simulink model "SA_asservissement_seul"  (R2016a)
settings: Solver=VariableStepAuto  StartTime=0.0  StopTime=5  RelTol=1e-3
values from neighbouring files (symbols this model uses):
  den_a_Z = [1 -p]    [SA_9.m]    (also in SA_global.m)
  den_AvPh = [1 -p]    [SA_global.m]
  den_PI = [1 -p]    [SA_global.m]
  den_r_Z = [1 -p_re]    [SA_9.m]    (also in SA_global.m)
  Ka_SA8 = abs((polyval(den_phi,pdes)*polyval(den_AvPh_SA8,pdes)*polyval(den_PI_SA8,pdes))/(polyval(num_AvPh_SA8,pdes)*polyval(num_phi,pdes)*polyval(num_PI_SA8,pdes)))    [SA_8.m]    (also in SA_global.m = abs((polyval(den_phi,pdes)*polyval(den_AvPh,pdes)*polyval(de)
  Kp_XX = -z*Kv_XX    [SA_10.m]    (also in SA_10x.m; SA_10y.m; SA_global.m)
  Kp_YY = -z*Kv_YY    [SA_10y.m]    (also in SA_global.m)
  Kv_XX = 1/abs(polyval(conv(num_a_XX,num_Sx(1,:)),p_des)/polyval(conv(den_a_XX,den_Sx),p_des))    [SA_10.m]    (also in SA_10x.m; SA_10y.m; SA_global.m)
  Kv_YY = 1/abs(polyval(conv(num_a_YY,num_Sy(1,:)),p_des)/polyval(conv(den_a_YY,den_Sy),p_des))    [SA_10y.m]    (also in SA_global.m)
  num_a_Z = Ka_Z*[1 -z]    [SA_9.m]    (also in SA_global.m)
  num_AvPh = [1 -z]    [SA_global.m]
  num_PI = [1 -z]    [SA_global.m]
  num_r_Z = [1 -z_re]    [SA_9.m]    (also in SA_global.m)
undefined symbols (not defined in the file or in its folder): A_theta, A_z, B_theta, B_z, C_theta, C_z, D_theta_1sortie, D_z_1sortie
settings Model: Creator=genp2203  LastModifiedBy=genp2203

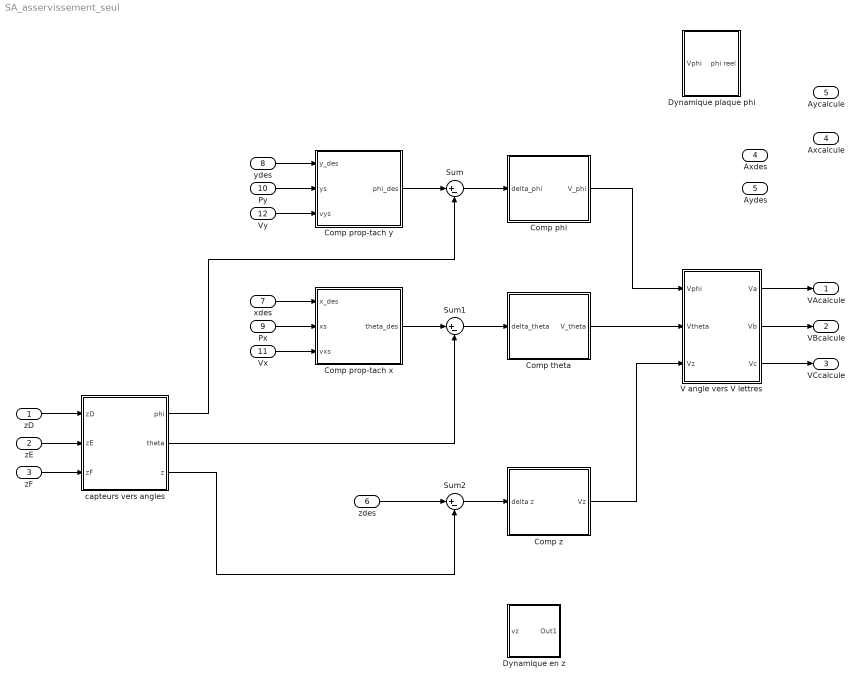
== system SA_asservissement_seul ==
  zD : Inport
  zE : Inport  Port=2
  zF : Inport  Port=3
  Axdes : Inport  Port=4
  Aydes : Inport  Port=5
  zdes : Inport  Port=6
  xdes : Inport  Port=7
  ydes : Inport  Port=8
  Px : Inport  Port=9
  Py : Inport  Port=10
  Vx : Inport  Port=11
  Vy : Inport  Port=12
  Comp phi : Subsystem
  Comp prop-tach x : Subsystem
  Comp prop-tach y : Subsystem
  Comp theta : Subsystem
  Comp z : Subsystem
  Dynamique en z : Subsystem
  Dynamique plaque phi : Subsystem
  Sum : Sum  Inputs=|+-
  Sum1 : Sum  Inputs=|+-
  Sum2 : Sum  Inputs=|+-
  V angle vers V lettres : Subsystem
  capteurs vers angles : Subsystem
  VAcalcule : Outport
  VBcalcule : Outport  Port=2
  VCcalcule : Outport  Port=3
  Axcalcule : Outport  Port=4
  Aycalcule : Outport  Port=5
  wires:
  Sum/1 -> Comp phi/1(delta_phi)
  ydes/1 -> Comp prop-tach y/1(y_des)
  xdes/1 -> Comp prop-tach x/1(x_des)
  Vx/1 -> Comp prop-tach x/3(vxs)
  Px/1 -> Comp prop-tach x/2(xs)
  Py/1 -> Comp prop-tach y/2(ys)
  Vy/1 -> Comp prop-tach y/3(vys)
  Comp prop-tach y/1(phi_des) -> Sum/1
  zD/1 -> capteurs vers angles/1(zD)
  zE/1 -> capteurs vers angles/2(zE)
  zF/1 -> capteurs vers angles/3(zF)
  capteurs vers angles/1(phi) -> Sum/2
  V angle vers V lettres/3(Vc) -> VCcalcule/1
  V angle vers V lettres/2(Vb) -> VBcalcule/1
  V angle vers V lettres/1(Va) -> VAcalcule/1
  Comp phi/1(V_phi) -> V angle vers V lettres/1(Vphi)
  Comp theta/1(V_theta) -> V angle vers V lettres/2(Vtheta)
  Comp prop-tach x/1(theta_des) -> Sum1/1
  Sum1/1 -> Comp theta/1(delta_theta)
  capteurs vers angles/2(theta) -> Sum1/2
  capteurs vers angles/3(z) -> Sum2/2
  zdes/1 -> Sum2/1
  Sum2/1 -> Comp z/1(delta z)
  Comp z/1(Vz) -> V angle vers V lettres/3(Vz)

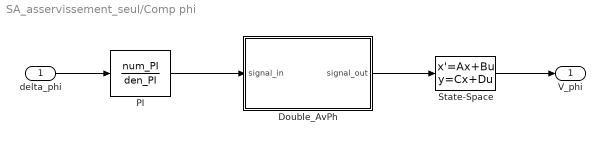
== system SA_asservissement_seul/Comp phi ==
  delta_phi : Inport
  Double_AvPh : Subsystem
  PI : TransferFcn  Numerator=num_PI  Denominator=den_PI
  State-Space : StateSpace  A=A_theta  B=B_theta  C=C_theta  D=D_theta_1sortie  X0=0
  V_phi : Outport
  wires:
  PI/1 -> Double_AvPh/1(signal_in)
  Double_AvPh/1(signal_out) -> State-Space/1
  State-Space/1 -> V_phi/1
  delta_phi/1 -> PI/1

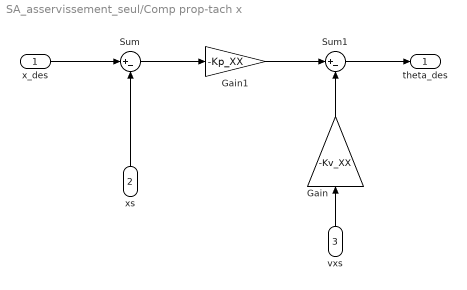
== system SA_asservissement_seul/Comp prop-tach x ==
  x_des : Inport
  xs : Inport  Port=2
  vxs : Inport  Port=3
  Gain : Gain  Gain=-Kv_XX
  Gain1 : Gain  Gain=-Kp_XX
  Sum : Sum  Inputs=|+-
  Sum1 : Sum  Inputs=|+-
  theta_des : Outport
  wires:
  Sum/1 -> Gain1/1
  x_des/1 -> Sum/1
  Gain1/1 -> Sum1/1
  Gain/1 -> Sum1/2
  xs/1 -> Sum/2
  vxs/1 -> Gain/1
  Sum1/1 -> theta_des/1

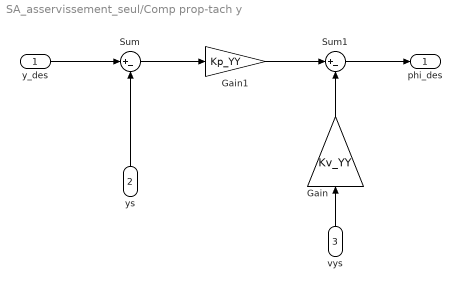
== system SA_asservissement_seul/Comp prop-tach y ==
  y_des : Inport
  ys : Inport  Port=2
  vys : Inport  Port=3
  Gain : Gain  Gain=Kv_YY
  Gain1 : Gain  Gain=Kp_YY
  Sum : Sum  Inputs=|+-
  Sum1 : Sum  Inputs=|+-
  phi_des : Outport
  wires:
  Sum/1 -> Gain1/1
  y_des/1 -> Sum/1
  Gain1/1 -> Sum1/1
  Gain/1 -> Sum1/2
  ys/1 -> Sum/2
  vys/1 -> Gain/1
  Sum1/1 -> phi_des/1

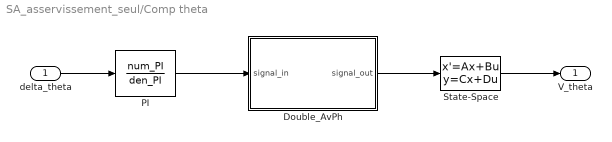
== system SA_asservissement_seul/Comp theta ==
  delta_theta : Inport
  Double_AvPh : Subsystem
  PI : TransferFcn  Numerator=num_PI  Denominator=den_PI
  State-Space : StateSpace  A=A_theta  B=B_theta  C=C_theta  D=D_theta_1sortie  X0=0
  V_theta : Outport
  wires:
  PI/1 -> Double_AvPh/1(signal_in)
  Double_AvPh/1(signal_out) -> State-Space/1
  State-Space/1 -> V_theta/1
  delta_theta/1 -> PI/1

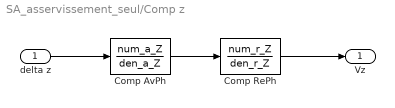
== system SA_asservissement_seul/Comp z ==
  delta z : Inport
  Comp AvPh : TransferFcn  Numerator=num_a_Z  Denominator=den_a_Z
  Comp RePh : TransferFcn  Numerator=num_r_Z  Denominator=den_r_Z
  Vz : Outport
  wires:
  Comp AvPh/1 -> Comp RePh/1
  Comp RePh/1 -> Vz/1
  delta z/1 -> Comp AvPh/1

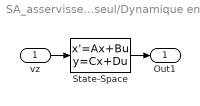
== system SA_asservissement_seul/Dynamique en z ==
  vz : Inport
  State-Space : StateSpace  A=A_z  B=B_z  C=C_z  D=D_z_1sortie  X0=0
  Out1 : Outport
  wires:
  vz/1 -> State-Space/1
  State-Space/1 -> Out1/1

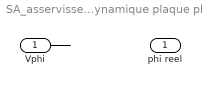
== system SA_asservissement_seul/Dynamique plaque phi ==
  Vphi : Inport
  phi reel : Outport
  wires:
  Vphi/1 -> ?
  ? -> phi reel/1

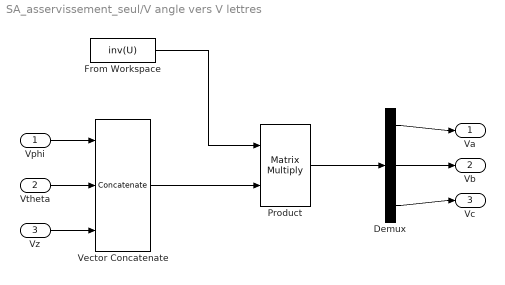
== system SA_asservissement_seul/V angle vers V lettres ==
  Vphi : Inport
  Vtheta : Inport  Port=2
  Vz : Inport  Port=3
  Demux : Demux  Outputs=3
  From Workspace : FromWorkspace  VariableName=inv(U)  SampleTime=0
  Product : Product  Multiplication=Matrix(*)
  Vector Concatenate : Concatenate  NumInputs=3  Mode=Multidimensional array
  Va : Outport
  Vb : Outport  Port=2
  Vc : Outport  Port=3
  wires:
  Vz/1 -> Vector Concatenate/3
  Vtheta/1 -> Vector Concatenate/2
  Vphi/1 -> Vector Concatenate/1
  Product/1 -> Demux/1
  From Workspace/1 -> Product/1
  Vector Concatenate/1 -> Product/2
  Demux/3 -> Vc/1
  Demux/2 -> Vb/1
  Demux/1 -> Va/1

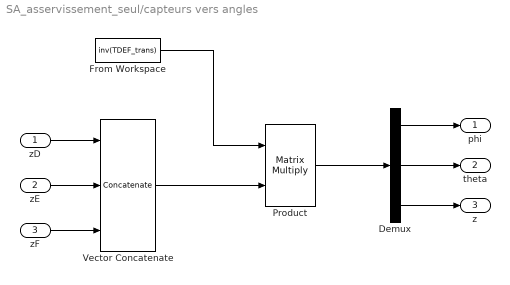
== system SA_asservissement_seul/capteurs vers angles ==
  zD : Inport
  zE : Inport  Port=2
  zF : Inport  Port=3
  Demux : Demux  Outputs=3
  From Workspace : FromWorkspace  VariableName=inv(TDEF_trans)  SampleTime=0
  Product : Product  Multiplication=Matrix(*)
  Vector Concatenate : Concatenate  NumInputs=3  Mode=Multidimensional array
  phi : Outport
  theta : Outport  Port=2
  z : Outport  Port=3
  wires:
  zF/1 -> Vector Concatenate/3
  zE/1 -> Vector Concatenate/2
  zD/1 -> Vector Concatenate/1
  Product/1 -> Demux/1
  From Workspace/1 -> Product/1
  Vector Concatenate/1 -> Product/2
  Demux/3 -> z/1
  Demux/2 -> theta/1
  Demux/1 -> phi/1

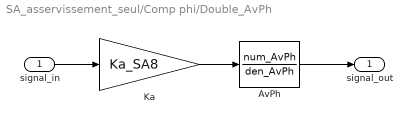
== system SA_asservissement_seul/Comp phi/Double_AvPh ==
  signal_in : Inport
  AvPh : TransferFcn  Numerator=num_AvPh  Denominator=den_AvPh
  Ka : Gain  Gain=Ka_SA8
  signal_out : Outport
  wires:
  signal_in/1 -> Ka/1
  Ka/1 -> AvPh/1
  AvPh/1 -> signal_out/1

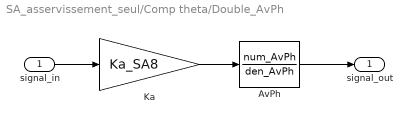
== system SA_asservissement_seul/Comp theta/Double_AvPh ==
  signal_in : Inport
  AvPh : TransferFcn  Numerator=num_AvPh  Denominator=den_AvPh
  Ka : Gain  Gain=Ka_SA8
  signal_out : Outport
  wires:
  signal_in/1 -> Ka/1
  Ka/1 -> AvPh/1
  AvPh/1 -> signal_out/1
